simulink model "chap02_02_57_mdl"  (R2013b)
settings: Solver=ode45  StartTime=0.0  StopTime=10.0  RelTol=1e-3
settings Model: Creator=Administrator  LastModifiedBy=sunzx.fnst

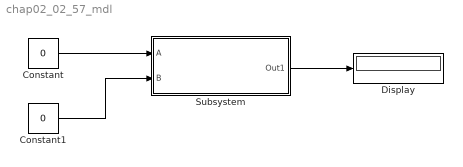
== system chap02_02_57_mdl ==
  Constant : Constant  Value=0
  Constant1 : Constant  Value=0
  Display : Display
  Subsystem : Subsystem
  wires:
  Subsystem/1(Out1) -> Display/1
  Constant1/1 -> Subsystem/2(B)
  Constant/1 -> Subsystem/1(A)

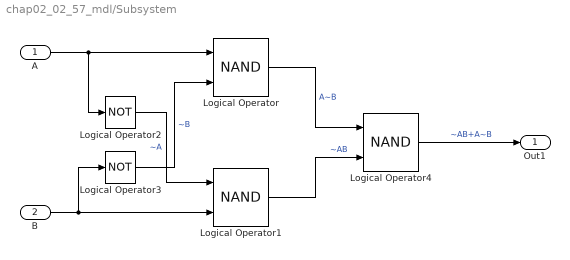
== system chap02_02_57_mdl/Subsystem ==
  A : Inport
  B : Inport  Port=2
  Logical Operator : Logic  Operator=NAND  IconShape=distinctive  AllPortsSameDT=off  OutDataTypeStr=boolean
  Logical Operator1 : Logic  Operator=NAND  IconShape=distinctive  AllPortsSameDT=off  OutDataTypeStr=boolean
  Logical Operator2 : Logic  Operator=NOT  IconShape=distinctive  AllPortsSameDT=off  OutDataTypeStr=boolean
  Logical Operator3 : Logic  Operator=NOT  IconShape=distinctive  AllPortsSameDT=off  OutDataTypeStr=boolean
  Logical Operator4 : Logic  Operator=NAND  IconShape=distinctive  AllPortsSameDT=off  OutDataTypeStr=boolean
  Out1 : Outport
  wires:
  Logical Operator1/1 -> Logical Operator4/2  "~AB"
  A/1 -> Logical Operator/1, Logical Operator2/1
  Logical Operator3/1 -> Logical Operator/2  "~B"
  Logical Operator2/1 -> Logical Operator1/1  "~A"
  B/1 -> Logical Operator3/1, Logical Operator1/2
  Logical Operator4/1 -> Out1/1  "~AB+A~B"
  Logical Operator/1 -> Logical Operator4/1  "A~B"
